simulink model "Manipulador_de_un_enlace"  (R2024a)
settings: Solver=VariableStepAuto  StartTime=0.0  StopTime=100  RelTol=1e-3
settings Model: Creator=ansm3  LastModifiedBy=ansm3

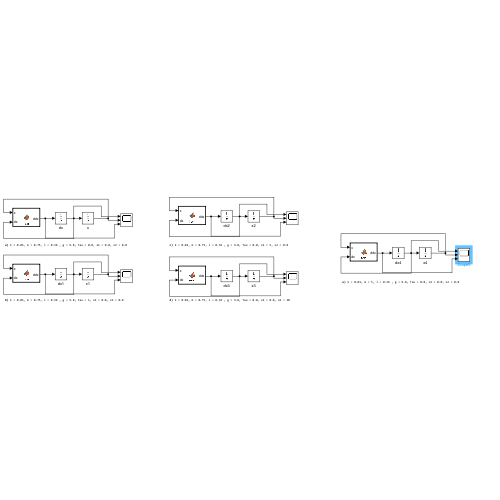
[thumbnail: Simulink's stored preview of the top-level diagram]
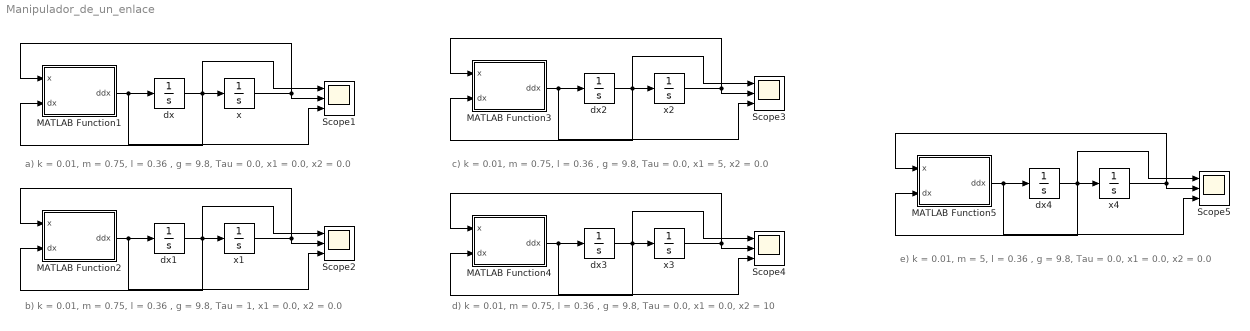
== system Manipulador_de_un_enlace ==
  note: a) k = 0.01, m = 0.75, l = 0.36 , g = 9.8, Tau = 0.0, x1 = 0.0, x2 = 0.0
  note: b) k = 0.01, m = 0.75, l = 0.36 , g = 9.8, Tau = 1, x1 = 0.0, x2 = 0.0
  note: c) k = 0.01, m = 0.75, l = 0.36 , g = 9.8, Tau = 0.0, x1 = 5, x2 = 0.0
  note: d) k = 0.01, m = 0.75, l = 0.36 , g = 9.8, Tau = 0.0, x1 = 0.0, x2 = 10
  note: e) k = 0.01, m = 5, l = 0.36 , g = 9.8, Tau = 0.0, x1 = 0.0, x2 = 0.0
  MATLAB Function1 : MATLAB Function  TreatAsAtomicUnit=on
  MATLAB Function2 : MATLAB Function  TreatAsAtomicUnit=on
  MATLAB Function3 : MATLAB Function  TreatAsAtomicUnit=on
  MATLAB Function4 : MATLAB Function  TreatAsAtomicUnit=on
  MATLAB Function5 : MATLAB Function  TreatAsAtomicUnit=on
  Scope{1..5} (5 alike) : Scope  NumInputPorts=3
  dx{,1..4} (5 alike) : Integrator  ContinuousStateAttributes="\"dx\""
  x{,1..4} (5 alike) : Integrator
  wires:
  dx/1 -> Scope1/1, MATLAB Function1/2(dx), x/1
  MATLAB Function1/1(ddx) -> Scope1/3, dx/1
  x/1 -> Scope1/2, MATLAB Function1/1(x)
  x1/1 -> Scope2/2, MATLAB Function2/1(x)
  MATLAB Function2/1(ddx) -> Scope2/3, dx1/1
  dx1/1 -> Scope2/1, MATLAB Function2/2(dx), x1/1
  dx2/1 -> Scope3/1, MATLAB Function3/2(dx), x2/1
  MATLAB Function3/1(ddx) -> Scope3/3, dx2/1
  x2/1 -> Scope3/2, MATLAB Function3/1(x)
  dx3/1 -> Scope4/1, MATLAB Function4/2(dx), x3/1
  MATLAB Function4/1(ddx) -> Scope4/3, dx3/1
  x3/1 -> Scope4/2, MATLAB Function4/1(x)
  dx4/1 -> Scope5/1, MATLAB Function5/2(dx), x4/1
  MATLAB Function5/1(ddx) -> Scope5/3, dx4/1
  x4/1 -> Scope5/2, MATLAB Function5/1(x)

== matlab function Manipulador_de_un_enlace/MATLAB Function2 ==
  data: x input; ddx output; dx input
function ddx = fcn(x, dx)

k=0.01;
l=0.36;
g=9.8;
a=l/2;

m=0.75;
J=(4/3)*(m*a^2);
tao=1;

x1=0.0+x;
x2=0.0+dx;

ddx=(1/J)*(tao-m*g*a*(cos(x1))-k*x2);

== matlab function Manipulador_de_un_enlace/MATLAB Function3 ==
  data: x input; ddx output; dx input
function ddx = fcn(x, dx)

k=0.01;
l=0.36;
g=9.8;
a=l/2;

m=0.75;
J=(4/3)*(m*a^2);
tao=0.0;

x1=5+x;
x2=0.0+dx;

ddx=(1/J)*(tao-m*g*a*(cos(x1))-k*x2);

== matlab function Manipulador_de_un_enlace/MATLAB Function4 ==
  data: x input; ddx output; dx input
function ddx = fcn(x, dx)

k=0.01;
l=0.36;
g=9.8;
a=l/2;

m=0.75;
J=(4/3)*(m*a^2);
tao=0.0;

x1=0.0+x;
x2=10+dx;

ddx=(1/J)*(tao-m*g*a*(cos(x1))-k*x2);

== matlab function Manipulador_de_un_enlace/MATLAB Function5 ==
  data: x input; ddx output; dx input
function ddx = fcn(x, dx)

k=0.01;
l=0.36;
g=9.8;
a=l/2;

m=5;
J=(4/3)*(m*a^2);
tao=0.0;

x1=0.0+x;
x2=0.0+dx;

ddx=(1/J)*(tao-m*g*a*(cos(x1))-k*x2);

== matlab function Manipulador_de_un_enlace/MATLAB Function1 ==
  data: x input; ddx output; dx input
function ddx = fcn(x, dx)

k=0.01;
l=0.36;
g=9.8;
a=l/2;

m=0.75;
J=(4/3)*(m*a^2);
tao=0.0;

x1=0.0+x;
x2=0.0+dx;

ddx=(1/J)*(tao-m*g*a*(cos(x1))-k*x2);
